simulink subsystem "PvtSubSys_LATC"  (R2020b)
settings: Solver=VariableStepAuto  StartTime=0.0  StopTime=10.0  RelTol=1e-3
values from neighbouring files (symbols this model uses):
  P_Global_CharSpd_ms : value not decoded    [PubParsGlobal.sldd]
  P_Global_SteeringAngleRatio : value not decoded    [PubParsGlobal.sldd]
  P_Global_WheelBase_m : value not decoded    [PubParsGlobal.sldd]
  P_LCS_A0_Limit = 0.25    [LATC.sldd]    (also in LCS_v05.sldd)
  P_LCS_A1_Limit = 0.002    [LATC.sldd]    (also in LCS_v05.sldd)
  P_LCS_communicationTest = 1.0    [LATC.sldd]    (also in LCS_v05.sldd)
  P_LCS_Current_Offset_Test_SW = 0.0    [LATC.sldd]
  P_LCS_Current_Offset_Test_Value = 0.0    [LATC.sldd]
  P_LCS_Curvature_bp : value not decoded    [LATC.sldd]
  P_LCS_CycleTime = 0.4 0.4 0.4 0.4 0.4 0.4 0.4 0.4 0.4 0.6 0.6 0.6 0.6 0.6 0.6 0.6 0.4 0.4 0.4 0.4 0.4 0.4 0.4 0.4 0.4 0.6 0.6 0.6 0.6 0.6 0.6 0.6 0.4 0.4 0.4 0.4 0.4 0.4 0.4 0.4 0.4 0.6 0.6 0.6 0.6 0.6 0.6 0.6 0.4 0.4 0.4 0.4 0.4 0.4 0.4 0.4 0.4 0.6 0.6 0.6 0.6 0.6 0.6 0.6 0.4 0.4 0.4 0.4 0.4 0.4 0.4 0.4 0.4 0.6 0.6 0.6 0.6 0.6 0.6 0.6 0.4 0.4 0.4 0.4 0.4 0.4 0.4 0.4 0.4 0.6 0.6 0.6 0.6 0.6 0.6 0.6 0.4 0.4 0.4 0.4    [LATC.sldd]
  P_LCS_ESS_AngleSlope_Limit = 2.9    [LATC.sldd]    (also in LCS_v05.sldd)
  P_LCS_IN_Offset_Test_SW = 0.0    [LATC.sldd]    (also in LCS_v05.sldd)
  P_LCS_IN_Offset_Test_Value = 0.0    [LATC.sldd]    (also in LCS_v05.sldd)
  P_LCS_LATC_CurOffsetVehicleSpdLimitValue_degs = 7.0    [LATC.sldd]
  P_LCS_LATC_Du_Max = 20.0    [LATC.sldd]
  P_LCS_LATC_ELKAngleSlope_ratio : value not decoded    [LATC.sldd]
  P_LCS_LATC_ELKMaxLatAcc_ms2 : value not decoded    [LATC.sldd]
  P_LCS_LATC_ESSAngleSlope_ratio : value not decoded    [LATC.sldd]
  P_LCS_LATC_ESSMaxLatAcc_ms2 : value not decoded    [LATC.sldd]
  P_LCS_LATC_LCAngleSlope_ratio : value not decoded    [LATC.sldd]
  P_LCS_LATC_LCCancleMaxLatAcc_ms2 : value not decoded    [LATC.sldd]
  P_LCS_LATC_LCEcoAngleSlope_ratio : value not decoded    [LATC.sldd]
  P_LCS_LATC_LCEcoMaxLatAcc_ms2 : value not decoded    [LATC.sldd]
  P_LCS_LATC_LCKAngleSlope_ratio : value not decoded    [LATC.sldd]
  P_LCS_LATC_LCKIEAngleSlope_ratio : value not decoded    [LATC.sldd]
  P_LCS_LATC_LCKIEMaxLatAcc_ms2 : value not decoded    [LATC.sldd]
  P_LCS_LATC_LCKMaxLatAcc_ms2 : value not decoded    [LATC.sldd]
  P_LCS_LATC_LCNormalAngleSlope_ratio : value not decoded    [LATC.sldd]
  P_LCS_LATC_LCNormalMaxLatAcc_ms2 : value not decoded    [LATC.sldd]
  P_LCS_LATC_LCSportAngleSlope_ratio : value not decoded    [LATC.sldd]
  P_LCS_LATC_LCSportMaxLatAcc_ms2 : value not decoded    [LATC.sldd]
  P_LCS_LATC_LKAAngleSlope_ratio : value not decoded    [LATC.sldd]
  P_LCS_LATC_LKAMaxLatAcc_ms2 : value not decoded    [LATC.sldd]
  P_LCS_LATC_MatrixQ1_st = 0.8 0.8 1.2 1.4 1.4 1.4 2.0 2.2 2.2 2.2 2.2 2.2 2.2 2.2 2.2 2.2 0.8 0.8 1.2 1.4 1.4 1.4 2.0 2.2 2.2 2.2 2.2 2.2 2.2 2.2 2.2 2.2 0.8 0.8 1.2 1.4 1.4 1.4 2.0 2.2 2.2 2.2 2.2 2.2 2.2 2.2 2.2 2.2 0.8 0.8 1.2 1.4 1.4 1.4 2.0 2.2 2.2 2.2 2.2 2.2 2.2 2.2 2.2 2.2 0.8 0.8 1.2 1.4 1.4 1.4 2.0 2.2 2.2 2.2 2.2 2.2 2.2 2.2 2.2 2.2 0.8 0.8 1.2 1.4 1.4 1.4 2.0 2.2 2.2 2.2 2.2 2.2 2.2 2.2 2.2 2.2 0.8 0.8 1.2 1.4    [LATC.sldd]
  P_LCS_LATC_MatrixQ3_st = 20.0 20.0 20.0 20.0 20.0 15.0 15.0 15.0 15.0 15.0 15.0 15.0 15.0 13.0 13.0 13.0 20.0 20.0 20.0 20.0 20.0 15.0 15.0 15.0 15.0 15.0 15.0 15.0 15.0 13.0 13.0 13.0 20.0 20.0 20.0 20.0 20.0 15.0 15.0 15.0 15.0 15.0 15.0 15.0 15.0 13.0 13.0 13.0 20.0 20.0 20.0 20.0 20.0 15.0 15.0 15.0 15.0 15.0 15.0 15.0 15.0 13.0 13.0 13.0 20.0 20.0 20.0 20.0 20.0 15.0 15.0 15.0 15.0 15.0 15.0 15.0 15.0 13.0 13.0 13.0    [LATC.sldd]
  P_LCS_LATC_MatrixR_st = 10.0 10.0 10.0 10.0 10.0 10.0 10.0 15.0 15.0 15.0 15.0 15.0 15.0 15.0 15.0 15.0 10.0 10.0 10.0 10.0 10.0 10.0 10.0 15.0 15.0 15.0 15.0 15.0 15.0 15.0 15.0 15.0 10.0 10.0 10.0 10.0 10.0 10.0 10.0 15.0 15.0 15.0 15.0 15.0 15.0 15.0 15.0 15.0 10.0 10.0 10.0 10.0 10.0 10.0 10.0 15.0 15.0 15.0 15.0 15.0 15.0 15.0 15.0 15.0 10.0 10.0 10.0 10.0 10.0 10.0 10.0 15.0 15.0 15.0 15.0 15.0 15.0 15.0 15.0 15.0    [LATC.sldd]
  P_LCS_LATC_Max_LatAcc = 4.0    [LATC.sldd]
  P_LCS_LATC_Max_Phi = 15.0    [LATC.sldd]
  P_LCS_LATC_Max_y = 0.5    [LATC.sldd]
  P_LCS_LATC_MPC_SW = 0.0    [LATC.sldd]
  P_LCS_LATC_PreView_SW = 1.0    [LATC.sldd]
  P_LCS_LATC_SoftConstWeight = 1.0    [LATC.sldd]
  P_LCS_LATC_StateActivAngleSlopeLimit_ratio : value not decoded    [LATC.sldd]
  P_LCS_LATC_StateActiveFlg_TabX_st : value not decoded    [LATC.sldd]
  P_LCS_LATC_StateActiveHoldTime_TabY_st : value not decoded    [LATC.sldd]
  P_LCS_LATC_StateHoldTime_st = 250.0    [LATC.sldd]
  P_LCS_LATC_TarAngleFliterWindowSize = 5.0    [LATC.sldd]
  P_LCS_LATC_TarAngleLP_Time = 0.02    [LATC.sldd]
  P_LCS_LATC_U_Max = 90.0    [LATC.sldd]
  P_LCS_LCK_AngleSlope_Limit = 1.4    [LATC.sldd]
  P_LCS_LineVaildSW = 0.0    [LATC.sldd]
  P_LCS_Lookahead_Distance : value not decoded    [LATC.sldd]
  P_LCS_Lookahead_DistanceFac : value not decoded    [LATC.sldd]
  P_LCS_PLAN_CurvePreView_s = 0.3    [LATC.sldd]
  P_LCS_PLAN_CurvePreview_TabX_m : value not decoded    [LATC.sldd]
  P_LCS_PLAN_CurvePreViewFilterTime_s = 0.1    [LATC.sldd]
  P_LCS_PLAN_ELKAyDtLimit_Tab_ms3 = 1.0 1.0 1.0 1.0 1.0 1.0 1.0 1.0 1.0 1.0 1.0 1.0 1.0 1.0 1.0 1.0 1.0 1.0 1.0 1.0 1.0 1.0 1.0 1.0 1.0 1.0 1.0 1.0 1.0 1.0 1.0 1.0 1.0 1.0 1.0 1.0 1.0 1.0 1.0 1.0 1.0 1.0 1.0 1.0 1.0 1.0 1.0 1.0 1.0 1.0 1.0 1.0 1.0 1.0 1.0 1.0 1.0 1.0 1.0 1.0 1.0 1.0 1.0 1.0 1.0 1.0 1.0 1.0 1.0 1.0 1.0 1.0 1.0 1.0 1.0 1.0 1.0 1.0 1.0 1.0 1.0 1.0 1.0 1.0 1.0 1.0 1.0 1.0 1.0 1.0 1.0 1.0 1.0 1.0 1.0 1.0 1.0 1.0 1.0 1.0    [LATC.sldd]
  P_LCS_PLAN_ESSAyDtLimit_Tab_ms3 = 1.0 1.0 1.0 1.0 1.0 1.0 1.0 1.0 1.0 1.0 1.0 1.0 1.0 1.0 1.0 1.0 1.0 1.0 1.0 1.0 1.0 1.0 1.0 1.0 1.0 1.0 1.0 1.0 1.0 1.0 1.0 1.0 1.0 1.0 1.0 1.0 1.0 1.0 1.0 1.0 1.0 1.0 1.0 1.0 1.0 1.0 1.0 1.0 1.0 1.0 1.0 1.0 1.0 1.0 1.0 1.0 1.0 1.0 1.0 1.0 1.0 1.0 1.0 1.0 1.0 1.0 1.0 1.0 1.0 1.0 1.0 1.0 1.0 1.0 1.0 1.0 1.0 1.0 1.0 1.0 1.0 1.0 1.0 1.0 1.0 1.0 1.0 1.0 1.0 1.0 1.0 1.0 1.0 1.0 1.0 1.0 1.0 1.0 1.0 1.0    [LATC.sldd]
  P_LCS_PLAN_LCCancleAyDtLimit_Tab_ms3 = 1.0 1.0 1.0 1.0 1.0 1.0 1.0 1.0 1.0 1.0 1.0 1.0 1.0 1.0 1.0 1.0 1.0 1.0 1.0 1.0 1.0 1.0 1.0 1.0 1.0 1.0 1.0 1.0 1.0 1.0 1.0 1.0 1.0 1.0 1.0 1.0 1.0 1.0 1.0 1.0 1.0 1.0 1.0 1.0 1.0 1.0 1.0 1.0 1.0 1.0 1.0 1.0 1.0 1.0 1.0 1.0 1.0 1.0 1.0 1.0 1.0 1.0 1.0 1.0 1.0 1.0 1.0 1.0 1.0 1.0 1.0 1.0 1.0 1.0 1.0 1.0 1.0 1.0 1.0 1.0 1.0 1.0 1.0 1.0 1.0 1.0 1.0 1.0 1.0 1.0 1.0 1.0 1.0 1.0 1.0 1.0 1.0 1.0 1.0 1.0    [LATC.sldd]
  P_LCS_PLAN_LCEcoAyDtLimit_Tab_ms3 = 1.0 1.0 1.0 1.0 1.0 1.0 1.0 1.0 1.0 1.0 1.0 1.0 1.0 1.0 1.0 1.0 1.0 1.0 1.0 1.0 1.0 1.0 1.0 1.0 1.0 1.0 1.0 1.0 1.0 1.0 1.0 1.0 1.0 1.0 1.0 1.0 1.0 1.0 1.0 1.0 1.0 1.0 1.0 1.0 1.0 1.0 1.0 1.0 1.0 1.0 1.0 1.0 1.0 1.0 1.0 1.0 1.0 1.0 1.0 1.0 1.0 1.0 1.0 1.0 1.0 1.0 1.0 1.0 1.0 1.0 1.0 1.0 1.0 1.0 1.0 1.0 1.0 1.0 1.0 1.0 1.0 1.0 1.0 1.0 1.0 1.0 1.0 1.0 1.0 1.0 1.0 1.0 1.0 1.0 1.0 1.0 1.0 1.0 1.0 1.0    [LATC.sldd]
  P_LCS_PLAN_LCKAyDtLimit_Tab_ms3 = 1.5 1.5 1.5 1.5 1.5 1.5 1.5 1.5 1.5 1.5 1.5 1.5 1.5 1.5 1.5 1.5 1.5 1.5 1.5 1.5 1.5 1.5 1.5 1.5 1.5 1.5 1.5 1.5 1.5 1.5 1.5 1.5 1.5 1.5 1.5 1.5 1.5 1.5 1.5 1.5 1.5 1.5 1.5 1.5 1.5 1.5 1.5 1.5 1.5 1.5 1.5 1.5 1.5 1.5 1.5 1.5 1.5 1.5 1.5 1.5 1.5 1.5 1.5 1.5 1.5 1.5 1.5 1.5 1.5 1.5 1.5 1.5 1.5 1.5 1.5 1.5 1.5 1.5 1.5 1.5 1.5 1.5 1.5 1.5 1.5 1.5 1.5 1.5 1.5 1.5 1.5 1.5 1.5 1.5 1.5 1.5 1.5 1.5 1.5 1.5    [LATC.sldd]
  P_LCS_PLAN_LCKIEAyDtLimit_Tab_ms3 = 1.0 1.0 1.0 1.0 1.0 1.0 1.0 1.0 1.0 1.0 1.0 1.0 1.0 1.0 1.0 1.0 1.0 1.0 1.0 1.0 1.0 1.0 1.0 1.0 1.0 1.0 1.0 1.0 1.0 1.0 1.0 1.0 1.0 1.0 1.0 1.0 1.0 1.0 1.0 1.0 1.0 1.0 1.0 1.0 1.0 1.0 1.0 1.0 1.0 1.0 1.0 1.0 1.0 1.0 1.0 1.0 1.0 1.0 1.0 1.0 1.0 1.0 1.0 1.0 1.0 1.0 1.0 1.0 1.0 1.0 1.0 1.0 1.0 1.0 1.0 1.0 1.0 1.0 1.0 1.0 1.0 1.0 1.0 1.0 1.0 1.0 1.0 1.0 1.0 1.0 1.0 1.0 1.0 1.0 1.0 1.0 1.0 1.0 1.0 1.0    [LATC.sldd]
  P_LCS_PLAN_LCNormalAyDtLimit_Tab_ms3 = 1.0 1.0 1.0 1.0 1.0 1.0 1.0 1.0 1.0 1.0 1.0 1.0 1.0 1.0 1.0 1.0 1.0 1.0 1.0 1.0 1.0 1.0 1.0 1.0 1.0 1.0 1.0 1.0 1.0 1.0 1.0 1.0 1.0 1.0 1.0 1.0 1.0 1.0 1.0 1.0 1.0 1.0 1.0 1.0 1.0 1.0 1.0 1.0 1.0 1.0 1.0 1.0 1.0 1.0 1.0 1.0 1.0 1.0 1.0 1.0 1.0 1.0 1.0 1.0 1.0 1.0 1.0 1.0 1.0 1.0 1.0 1.0 1.0 1.0 1.0 1.0 1.0 1.0 1.0 1.0 1.0 1.0 1.0 1.0 1.0 1.0 1.0 1.0 1.0 1.0 1.0 1.0 1.0 1.0 1.0 1.0 1.0 1.0 1.0 1.0    [LATC.sldd]
  P_LCS_PLAN_LCSportAyDtLimit_Tab_ms3 = 1.0 1.0 1.0 1.0 1.0 1.0 1.0 1.0 1.0 1.0 1.0 1.0 1.0 1.0 1.0 1.0 1.0 1.0 1.0 1.0 1.0 1.0 1.0 1.0 1.0 1.0 1.0 1.0 1.0 1.0 1.0 1.0 1.0 1.0 1.0 1.0 1.0 1.0 1.0 1.0 1.0 1.0 1.0 1.0 1.0 1.0 1.0 1.0 1.0 1.0 1.0 1.0 1.0 1.0 1.0 1.0 1.0 1.0 1.0 1.0 1.0 1.0 1.0 1.0 1.0 1.0 1.0 1.0 1.0 1.0 1.0 1.0 1.0 1.0 1.0 1.0 1.0 1.0 1.0 1.0 1.0 1.0 1.0 1.0 1.0 1.0 1.0 1.0 1.0 1.0 1.0 1.0 1.0 1.0 1.0 1.0 1.0 1.0 1.0 1.0    [LATC.sldd]
  P_LCS_PLAN_LKAAyDtLimit_Tab_ms3 = 1.0 1.0 1.0 1.0 1.0 1.0 1.0 1.0 1.0 1.0 1.0 1.0 1.0 1.0 1.0 1.0 1.0 1.0 1.0 1.0 1.0 1.0 1.0 1.0 1.0 1.0 1.0 1.0 1.0 1.0 1.0 1.0 1.0 1.0 1.0 1.0 1.0 1.0 1.0 1.0 1.0 1.0 1.0 1.0 1.0 1.0 1.0 1.0 1.0 1.0 1.0 1.0 1.0 1.0 1.0 1.0 1.0 1.0 1.0 1.0 1.0 1.0 1.0 1.0 1.0 1.0 1.0 1.0 1.0 1.0 1.0 1.0 1.0 1.0 1.0 1.0 1.0 1.0 1.0 1.0 1.0 1.0 1.0 1.0 1.0 1.0 1.0 1.0 1.0 1.0 1.0 1.0 1.0 1.0 1.0 1.0 1.0 1.0 1.0 1.0    [LATC.sldd]
  P_LCS_PLAN_MinPlanDis_m : value not decoded    [LATC.sldd]
  P_LCS_PLAN_PreCurMinDisFac_ratio : value not decoded    [LATC.sldd]
  P_LCS_PLAN_PreDisCurve_TabX_m : value not decoded    [LATC.sldd]
  P_LCS_PLAN_StateActiv_AyDtLimit_ms3 : value not decoded    [LATC.sldd]
  P_LCS_PLAN_VehicleSpd_TabX_kph : value not decoded    [LATC.sldd]
  P_LCS_PLAN_VehicleSpd_TabY_Kph : value not decoded    [LATC.sldd]
  P_LCS_Trq_Switch = 0.0    [LATC.sldd]    (also in LCS_v05.sldd)
  P_LCS_VehicleSpd_TabX_Kph : value not decoded    [LATC.sldd]
undefined symbols (not defined in the file or in its folder): HWP_AngCmdReqVal, HWP_AngCmdReqValVld, HWP_FuncTrqCmdReqFlag, HWP_ReqCtrlEPS, HWP_ReqCtrlEPSVld, HWP_TrqOvlCmdReqValue, HWP_WorkReq, HWP_WorkReqVld
libraries: simulink x4, dspbuff3 x2
(part 8 of 8)

== matlab function PvtSubSys_LATC/LATC/LateralControl/LCS_Angle/Controller/Understeer&Offset_Calc/YOD_Ackman ==
  data: AckConst output; VxvRef input; Vch input; WheelBase input; AlpWheelAngle input; PsiDtAckK1 input single; PsiDtAck output
function [AckConst,PsiDtAck] = Ackman(VxvRef,Vch,WheelBase,AlpWheelAngle,PsiDtAckK1)
%#codegen
if VxvRef==uint8(0)%转换常数数据类型
    PsiDtAckRaw = single(0);%转换常数数据类型
    AckConst = single(1);%转换常数数据类型
else
    AckConst = min((single(1)+VxvRef*VxvRef/(Vch*Vch))*WheelBase/VxvRef,single(32767));%转换常数数据类型
    PsiDtAckRaw = AlpWheelAngle/AckConst;
end
PsiDtAck = (single(0.02/0.1))*(PsiDtAckRaw-PsiDtAckK1)+PsiDtAckK1;%转换常数数据类型

== matlab function PvtSubSys_LATC/communicationTest4/MATLAB Function23 ==
  data: booleanoutk1 input boolean; booleanout output boolean; countk1 input uint8; count output uint8
function [booleanout,count] = boolean(booleanoutk1,countk1)
count=countk1+uint8(1);
booleanout=booleanoutk1;
if count>=100
    count=uint8(0);
end
if count==99
    if booleanoutk1==true
        booleanout=false;
    else
        booleanout=true;
    end
end

== matlab function PvtSubSys_LATC/LATC/LateralControl/LCS_Angle/Controller/TargetAngleCalc/SteerAngSlopeCalc/MATLAB Function3 ==
  data: delytime input uint16; TarDangerLevel input uint8; TarDangerLevelK1 input uint8; FLg output uint8; FLgK1 input uint8; CntK1 input uint16; Cnt output uint16
function [FLg,Cnt] = AngSlopeCalc(delytime,TarDangerLevel,TarDangerLevelK1,FLgK1,CntK1)

Cnt = min(CntK1 + uint16(1),delytime);
if Cnt== delytime
    FLg = uint8(0);
else
    FLg = FLgK1;
end
%FLg = FLgK1;
%% 
if TarDangerLevel==uint8(1) && TarDangerLevelK1==0  % NO function 2 LCK (TarDangerLevelK1==0)
    Cnt =uint16(0);
    FLg = uint8(1);
end

if  TarDangerLevel==uint8(3) && (TarDangerLevelK1==uint8(1)||TarDangerLevelK1==uint8(2)) % LCK/IE 2 LC_Normal
    Cnt =uint16(0);
    FLg = uint8(2);
end

if  TarDangerLevel==uint8(7) && (TarDangerLevelK1==uint8(1)||TarDangerLevelK1==uint8(2)) % LCK/IE 2 LC_Eco
    Cnt =uint16(0);
    FLg = uint8(3);
end

if  TarDangerLevel==uint8(8) && (TarDangerLevelK1==uint8(1)||TarDangerLevelK1==uint8(2)) % LCK/IE 2 LC_sport
    Cnt =uint16(0);
    FLg = uint8(4);
end
if  TarDangerLevel==uint8(6) && (TarDangerLevelK1==uint8(1)||TarDangerLevelK1==uint8(2)) % LCK/IE 2 ESS 后期添加配和ESS Slope 一起调试
    Cnt =uint16(0);
    FLg = uint8(5);
end

== matlab function PvtSubSys_LATC/communicationTest2/MATLAB Function7 ==
  data: factor input single; singlemin input single; singlemax input single; singleoutK1 input single; singleout output single; countk1 input uint8; count output uint8
function [singleout,count] = single(factor,singlemin,singlemax,singleoutK1,countk1)
count=countk1+uint8(1);
singleout=singleoutK1;
if count>=100
    count=uint8(0);
end
if count==99
    singleout=singleoutK1+factor;
    if singleout>singlemax
        singleout=singlemin;
    end      
end

== matlab function PvtSubSys_LATC/communicationTest/MATLAB Function19 ==
  data: uint8outK1 input uint8; uint8out output uint8; countk1 input uint8; count output uint8
function [uint8out,count] = uint8(uint8outK1,countk1)
count=countk1+uint8(1);
uint8out=uint8outK1;
if count>=100
    count=uint8(0);
end
if count==99
    uint8out=uint8outK1+uint8(1);
    if uint8out>2
        uint8out=uint8(0);
    end      
end

== matlab function PvtSubSys_LATC/LATC/LateralControl/LCS_Angle/Trajectory_Points/RoadCreate/MATLAB Function2 ==
  data: Veh_Speed input; A0 input size=[1 1]; Trajectory_x output; A1 input size=[1 1]; A2 input size=[1 1]; A3 input size=[1 1]; Trajectory_y output; numTraj output; AyDtLimit input; Min_Plan_Dis input; TrajPt output
function [Trajectory_x,Trajectory_y,numTraj,TrajPt]= LineDiscrete(Veh_Speed,A0,A1,A2,A3,AyDtLimit,Min_Plan_Dis)
rx1 = [single(0):single(1):single(9)]';  
rx2 = [single(10):10:150]';
rx = cat(1,rx1,rx2);
ry = A0 + A1.* rx + A2.* (rx.^2) + A3.* (rx.^3);
%创建路径点集合
waypoints = [rx,ry]; 
GtNumTrajpoints = single(150);
persistent referencePath
if isempty(referencePath)
    referencePath = FrenentReferencePath(GtNumTrajpoints);
end
referencePath.generationCartesianStates(waypoints,GtNumTrajpoints);
%% 定义轨迹起始点状态
initGlobalState = [0 0 0 0 Veh_Speed  0]; %暂时定义纵向加速度为0，[x, y,theta, kappa speed，Acc]
initFrenetState = referencePath.global2frenet(initGlobalState);
Pt = single([1.5 2 2.5 3 3.6 4.2 5 5.8 6.4 7 7.8 8.6 9.5 10.4 11.4]);
TarEgoAx = zeros(1,length(Pt));% 终点处期望纵向加速度
TarEgoV = ones(1,length(Pt)) .* Veh_Speed;% 终点处期望纵向速度
FtNumTarpoints = single(100);
persistent Frenet_traj_obj
if isempty(Frenet_traj_obj)
    Frenet_traj_obj = TrajectoryGeneratorFrenet(FtNumTarpoints);
end
%% 生成轨迹
for i = 1:length(Pt)
    Ps = round(1.05*(max(Veh_Speed,5)*Pt(i)));
    pathend= referencePath.interpolate(Ps);
    EndGlobalState = [pathend(1:4) TarEgoV(i) TarEgoAx(i)];
    EndFrenetState = referencePath.global2frenet(EndGlobalState);
    [frenetTrajectory,globalTrajectory] = Frenet_traj_obj.FrenetTrajectory...
        (referencePath,initFrenetState,EndFrenetState(1,1),0,EndFrenetState(1,2:3),EndFrenetState(1,5:6),Pt(i),FtNumTarpoints);
    AyDt = abs(diff(globalTrajectory.Trajectory(:,4).*((globalTrajectory.Trajectory(:,5).^2)))./diff(globalTrajectory.Times));
    if all(abs(AyDt) < AyDtLimit) && (frenetTrajectory.Trajectory(end,1) > Min_Plan_Dis)
        break;
    end
end

numTraj  = i;%借用numTraj输出时间点索引号
TrajPt = Pt(i);
[globalTrajectory] = EvaluateTrajectory(frenetTrajectory,globalTrajectory,1,0,1,1);
Trajectory_x = globalTrajectory(1).Trajectory(1:FtNumTarpoints,1);
Trajectory_y = globalTrajectory(1).Trajectory(1:FtNumTarpoints,2);
end

== matlab function PvtSubSys_LATC/LATC/LateralControl/LCS_Angle/Trajectory_Points/RoadCreate/Subsystem/MATLAB Function ==
  data: Forward_PreViewT input; VehSpd input; PreCurve output; C2 input; C3 input; PreCurve_Abs output
function [PreCurve,PreCurve_Abs]= PreView_Point_Curvature(Forward_PreViewT,VehSpd,C2,C3)
LookForwardDis = VehSpd * Forward_PreViewT;
PreCurve = 6*C3*LookForwardDis + 2*C2;
PreCurve_Abs = abs(PreCurve);
end
